simulink model "example"  (R2024b)
settings: Solver=FixedStepAuto  StartTime=0.0  StopTime=runT  FixedStep=1e-6  MaxStep=1e-6  RelTol=1e-3
InitFcn:
  | t_test = 1.14;
undefined symbols (not defined in the file or in its folder): injA, injF, injM, injT
libraries: simulink x1
settings Model: Creator=48926  LastModifiedBy=Daiiqi
settings DataIOCC: SignalLogging=off  DSMLogging=off  SaveTime=off  ReturnWorkspaceOutputs=off
settings ModelReferenceCC: EnableRefExpFcnMdlSchedulingChecks=on
settings RTWCC: GPUComputeCapability=3.5

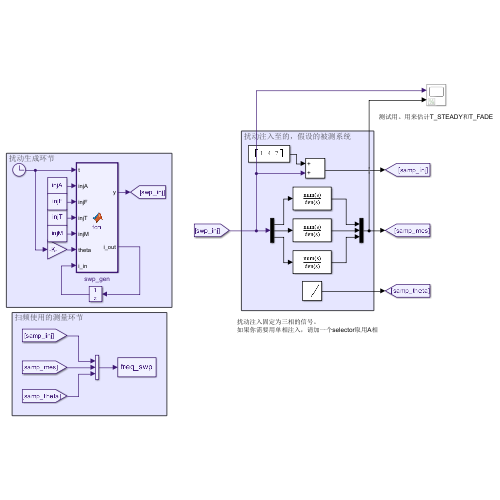
[thumbnail: Simulink's stored preview of the top-level diagram]
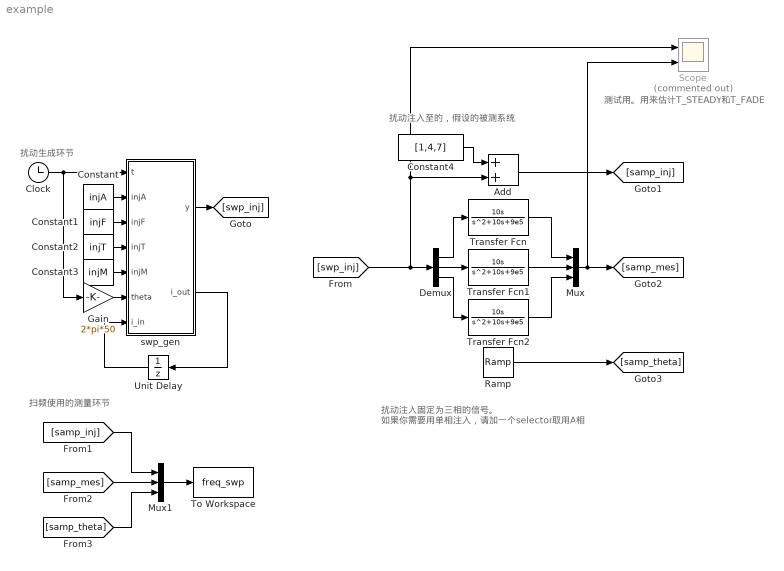
== system example ==
  note: 扫频使用的测量环节
  note: 扰动生成环节
  note: 扰动注入至的，假设的被测系统
  note: 扰动注入固定为三相的信号。
      | 如果你需要用单相注入，请加一个selector取用A相
  note: 测试用。用来估计T_STEADY和T_FADE
  Add : Sum
  Clock : Clock
  Constant : Constant  Value=injA
  Constant1 : Constant  Value=injF
  Constant2 : Constant  Value=injT
  Constant3 : Constant  Value=injM
  Constant4 : Constant  Value=[1,4,7]
  Demux : Demux  Outputs=3
  Gain : Gain  Gain=2*pi*50
  Mux : Mux  Inputs=3
  Mux1 : Mux  Inputs=3
  Ramp : simulink/Sources/Ramp  slope=2*50*pi  start=0  InitialOutput=0
  Scope : Scope  Commented=on  NumInputPorts=2
  To Workspace : ToWorkspace  VariableName=freq_swp  SaveFormat=Structure With Time  SampleTime=-1
  Transfer Fcn : TransferFcn  Numerator=[10, 0]  Denominator=[1, 10, 9e5]
  Transfer Fcn1 : TransferFcn  Numerator=[10, 0]  Denominator=[1, 10, 9e5]
  Transfer Fcn2 : TransferFcn  Numerator=[10, 0]  Denominator=[1, 10, 9e5]
  Unit Delay : UnitDelay  InitialCondition=1  SampleTime=-1  HasFrameUpgradeWarning=on
  swp_gen : MATLAB Function  TreatAsAtomicUnit=on
  wires:
  Clock/1 -> swp_gen/1(t), Gain/1
  Constant/1 -> swp_gen/2(injA)
  Constant1/1 -> swp_gen/3(injF)
  Constant2/1 -> swp_gen/4(injT)
  Constant3/1 -> swp_gen/5(injM)
  swp_gen/2(i_out) -> Unit Delay/1
  Unit Delay/1 -> swp_gen/7(i_in)
  Gain/1 -> swp_gen/6(theta)
  Demux/1 -> Transfer Fcn/1
  Demux/2 -> Transfer Fcn1/1
  Constant4/1 -> Add/1
  Ramp/1 -> [samp_theta]
  Mux1/1 -> To Workspace/1
  [samp_theta] -> Mux1/3
  swp_gen/1(y) -> [swp_inj]
  Add/1 -> [samp_inj]
  Demux/3 -> Transfer Fcn2/1
  [samp_inj] -> Mux1/1
  [samp_mes] -> Mux1/2
  [swp_inj] -> Scope/1, Add/2, Demux/1
  Transfer Fcn1/1 -> Mux/2
  Transfer Fcn2/1 -> Mux/3
  Transfer Fcn/1 -> Mux/1
  Mux/1 -> Scope/2, [samp_mes]

== matlab function example/swp_gen ==
  data: t input; y output; injA input; injF input; injT input; injM input; theta input; i_in input; i_out output
function [y, i_out] = fcn(t, injA, injF, injT, injM, theta, i_in)
%   t (1x1 double) 当前运行时刻
%   injA (NxM double) 小信号扰动源的幅值，N为时域关键帧数，M为同时的扫频点数
%   injF (NxM double) 小信号扰动源的频率
%   injT (Nx1 double) 小信号扰动源开始作用的时间帧
%   injM (Nx1 int32) 注入模式
%   i_in (1x1) 上一拍的"行"号

% 注意：矩阵[1,2,3; 4,5,6; 7,8,9]输入matlab function block时，会被自动变成列向量[1;4;7;2;5;8;3;6;9]。
% 所以这里的编程都按照对原矩阵取值的思路，变换到列向量下进行。
% 比如，对N行M列的矩阵，它原本的 (i,j) 会被映射到索引 (j-1)*N+i

N = numel(injT);
M = numel(injF)/N;

% 确定当前"行"号
if (i_in+1 <= N && t>=injT(i_in+1))
    i = i_in + 1;
else
    i = i_in;
end
i_out = i;

% 生成输出信号
y = zeros(3,1);
switch injM(i)
    case 0
        % P1
        for j = 1:M
            if injF((j-1)*N+i) == 0
                break
            else
                y(1) = y(1) + injA((j-1)*N+i) * cos(2*pi*injF((j-1)*N+i)*t);
            end
        end
    case 2
        % P3_a
        alpha = 0;
        for j = 1:M
            if injF((j-1)*N+i) == 0
                break
            else
                alpha = alpha + injA((j-1)*N+i) * cos(2*pi*injF((j-1)*N+i)*t);
            end
        end
        y(1) = sqrt(2/3) * alpha;
        y(2) = -sqrt(1/6) * alpha;
        y(3) = y(2);
    case 3
        % P3_b
        beta = 0;
        for j = 1:M
            if injF((j-1)*N+i) == 0
                break
            else
                beta = beta + injA((j-1)*N+i) * cos(2*pi*injF((j-1)*N+i)*t);
            end
        end
        y(1) = 0;
        y(2) = sqrt(1/2) * beta;
        y(3) = -y(2);
    case 5
        % P3_d
        d = 0;
        for j = 1:M
            if injF((j-1)*N+i) == 0
                break
            else
                d = d + injA((j-1)*N+i) * cos(2*pi*injF((j-1)*N+i)*t);
            end
        end
        y(1) = cos(theta) * d;
        y(2) = cos(theta - 2/3*pi) * d;
        y(3) = cos(theta + 2/3*pi) * d;
        y = sqrt(2/3) * y;
    case 6
        % P3_q
        q = 0;
        for j = 1:M
            if injF((j-1)*N+i) == 0
                break
            else
                q = q + injA((j-1)*N+i) * cos(2*pi*injF((j-1)*N+i)*t);
            end
        end
        y(1) = sin(theta) * q;
        y(2) = sin(theta - 2/3*pi) * q;
        y(3) = sin(theta + 2/3*pi) * q;
        y = -sqrt(2/3) * y;
    case 7
        % P3_pn
        for j = 1:M
            if injF((j-1)*N+i) == 0
                break
            else
                y(1) = y(1) + injA((j-1)*N+i) * cos(2*pi*injF((j-1)*N+i)*t);
                y(2) = y(2) + injA((j-1)*N+i) * cos(2*pi*injF((j-1)*N+i)*t - pi*2/3);
                y(3) = y(3) + injA((j-1)*N+i) * cos(2*pi*injF((j-1)*N+i)*t + pi*2/3);
            end
        end
end
